simulink library "inp"  (R2021b)
settings: Solver=VariableStepAuto  StartTime=0.0  StopTime=10.0  RelTol=1e-3
undefined symbols (not defined in the file): C_TASK_5MS_S, FALSE, KINP_AcoreReadyToSlp_flg_ovrdflg, KINP_AcoreReadyToSlp_flg_ovrdval, KINP_AllowMovThd_OTA_enum_ovrdflg, KINP_AllowMovThd_OTA_enum_ovrdval, KINP_APSAngleTarget_Deg_ovrdflg, KINP_APSAngleTarget_Deg_ovrdval, KINP_APSDecReq_mps2_ovrdflg, KINP_APSDecReq_mps2_ovrdval, KINP_APSDecReqA_flg_ovrdflg, KINP_APSDecReqA_flg_ovrdval, KINP_APSDFLL_cm_ovrdflg, KINP_APSDFLL_cm_ovrdval, KINP_APSDFLR_cm_ovrdflg, KINP_APSDFLR_cm_ovrdval, KINP_APSDRLL_cm_ovrdflg, KINP_APSDRLL_cm_ovrdval, KINP_APSDRLR_cm_ovrdflg, KINP_APSDRLR_cm_ovrdval, KINP_APSExitCondition_enum_ovrdflg, KINP_APSExitCondition_enum_ovrdval, KINP_APSHWVer_enum_ovrdflg, KINP_APSHWVer_enum_ovrdval, KINP_APSProgressPCT_pct_ovrdflg, KINP_APSProgressPCT_pct_ovrdval, KINP_APSPwrReq_enum_ovrdflg, KINP_APSPwrReq_enum_ovrdval, KINP_APSReq_enum_ovrdflg, KINP_APSReq_enum_ovrdval, KINP_APSRQDisplay_enum_ovrdflg, KINP_APSRQDisplay_enum_ovrdval, KINP_APSRqEPASCtrl_flg_ovrdflg, KINP_APSRqEPASCtrl_flg_ovrdval, KINP_APSShiftPosnReq_enum_ovrdval, KINP_APSShiftPosnReq_enum_ovrflg, KINP_APSSpeedCMD_kph_ovrdval, KINP_APSSpeedCMD_kph_ovrflg, KINP_APSStaSystem_enum_ovrdflg, KINP_APSStaSystem_enum_ovrdval, KINP_APSSWVer_enum_ovrdflg, KINP_APSSWVer_enum_ovrdval, KINP_APSVMCReqA_flg_ovrdval, KINP_APSVMCReqA_flg_ovrflg, KINP_APSVRqEPASCtrl_flg_ovrdflg, KINP_APSVRqEPASCtrl_flg_ovrdval, KINP_AuxBattVolmV_mV_ovrdflg, KINP_AuxBattVolmV_mV_ovrdval, KINP_CAASSta_enum_ovrdflg, KINP_CAASSta_enum_ovrdval, KINP_CAASVMCReqA_flg_ovrdval, KINP_CAASVMCReqA_flg_ovrflg, KINP_CAN1BusOff_flg_ovrdflg, KINP_CAN1BusOff_flg_ovrdval, KINP_CAN2BusOff_flg_ovrdflg, KINP_CAN2BusOff_flg_ovrdval, KINP_CAN3BusOff_flg_ovrdflg, KINP_CAN3BusOff_flg_ovrdval, KINP_CAN4BusOff_flg_ovrdflg, KINP_CAN4BusOff_flg_ovrdval ... (+152)
libraries: FVT_lib x1035, hcu_lib x1
(part 8 of 33)

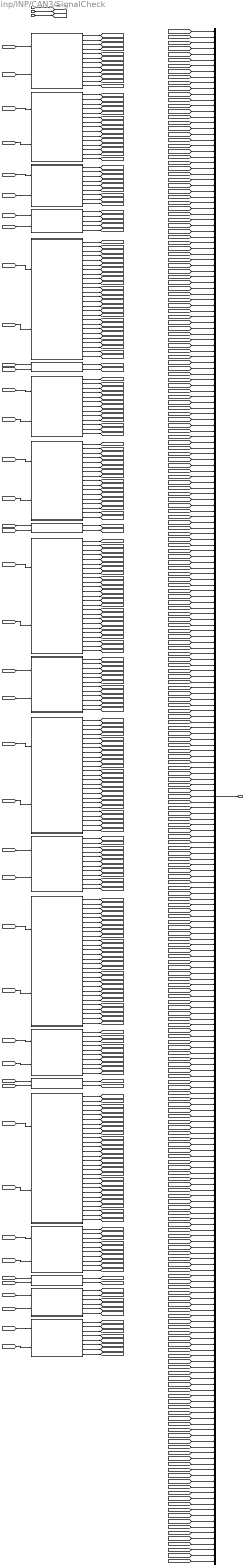
== system inp/INP/CAN3/SignalCheck ==
  inp_CanValid_bus : Inport
  TASK_TIME_S : Inport  Port=2
  BHAL_outputs : Inport  Port=3
  BMS1 : Subsystem
  BMS3 : Subsystem
  BMS4 : Subsystem
  BMS5 : Subsystem
  BMS6 : Subsystem
  BMS8 : Subsystem
  CCU1 : Subsystem
  CCU2 : Subsystem
  EBM1 : Subsystem
  MCU_B_F1 : Subsystem
  MCU_B_F2 : Subsystem
  MCU_B_R1 : Subsystem
  MCU_B_R2 : Subsystem
  MCU_N_F1 : Subsystem
  MCU_N_F2 : Subsystem
  MCU_N_F3 : Subsystem
  MCU_N_R1 : Subsystem
  MCU_N_R2 : Subsystem
  MCU_N_R3 : Subsystem
  Shifter1 : Subsystem
  Shifter2 : Subsystem
  bus_creator : BusCreator  Inputs=269
  inp_Hal_bus : Outport
  wires:
  inp_CanValid_bus/1 -> [inp_CanValid_bus]
  TASK_TIME_S/1 -> [TASK_TIME_S]
  BHAL_outputs/1 -> [BHAL_outputs]
  [BHAL_outputs] -> BMS1/1(BHAL_outputs)
  [inp_CanValid_bus] -> BMS1/2(inp_CanValid_bus)
  BMS1/1(VINP_BMS1CSErr_flg) -> [VINP_BMS1CSErr_flg]
  BMS1/2(VINP_BMS1RCErr_flg) -> [VINP_BMS1RCErr_flg]
  BMS1/3(VINP_BMSChckSum1_enum) -> [VINP_BMSChckSum1_enum]
  BMS1/4(VINP_BMSRolCnct1_enum) -> [VINP_BMSRolCnct1_enum]
  BMS1/5(VINP_HVBPwrAvailChrg_kW) -> [VINP_HVBPwrAvailChrg_kW]
  BMS1/6(VINP_HVBPwrAvailChrg30_kW) -> [VINP_HVBPwrAvailChrg30_kW]
  BMS1/7(VINP_HVBPwrAvailChrg60_kW) -> [VINP_HVBPwrAvailChrg60_kW]
  BMS1/8(VINP_HVBPwrAvailDchrg_kW) -> [VINP_HVBPwrAvailDchrg_kW]
  BMS1/9(VINP_HVBPwrAvailDchrg30_kW) -> [VINP_HVBPwrAvailDchrg30_kW]
  BMS1/10(VINP_HVBPwrAvailDchrg60_kW) -> [VINP_HVBPwrAvailDchrg60_kW]
  BMS1/11(VINP_HVBattCurr_A) -> [VINP_HVBattCurr_A]
  BMS1/12(VINP_HVBattVolt_V) -> [VINP_HVBattVolt_V]
  [BHAL_outputs] -> BMS3/1(BHAL_outputs)
  [inp_CanValid_bus] -> BMS3/2(inp_CanValid_bus)
  BMS3/1(VINP_ACChrgCurrDis_A) -> [VINP_ACChrgCurrDis_A]
  BMS3/2(VINP_FireDetErr_flg) -> [VINP_FireDetErr_flg]
  BMS3/3(VINP_HVBChrgPwr_kWh) -> [VINP_HVBChrgPwr_kWh]
  BMS3/4(VINP_HVBChrgPwrTotal_kWh) -> [VINP_HVBChrgPwrTotal_kWh]
  BMS3/5(VINP_HVBDrvPwr_kWh) -> [VINP_HVBDrvPwr_kWh]
  BMS3/6(VINP_HVBDrvPwrTotal_kWh) -> [VINP_HVBDrvPwrTotal_kWh]
  BMS3/7(VINP_HVBFullChrgPwr_kWh) -> [VINP_HVBFullChrgPwr_kWh]
  BMS3/8(VINP_HVBIsoImpedenceN_Megaohm) -> [VINP_HVBIsoImpedenceN_Megaohm]
  BMS3/9(VINP_HVBIsoImpedenceP_Megaohm) -> [VINP_HVBIsoImpedenceP_Megaohm]
  BMS3/10(VINP_HVBSOH_pct) -> [VINP_HVBSOH_pct]
  BMS3/11(VINP_HVBattErr_flg) -> [VINP_HVBattErr_flg]
  BMS3/12(VINP_HVBattPackVolt_V) -> [VINP_HVBattPackVolt_V]
  BMS3/13(VINP_HVBattSOC_pct) -> [VINP_HVBattSOC_pct]
  BMS3/14(VINP_HVBattSOCDis_pct) -> [VINP_HVBattSOCDis_pct]
  BMS3/15(VINP_RemainChrgTime_min) -> [VINP_RemainChrgTime_min]
  [BHAL_outputs] -> BMS4/1(BHAL_outputs)
  [inp_CanValid_bus] -> BMS4/2(inp_CanValid_bus)
  BMS4/1(VINP_CellTempAvg_C) -> [VINP_CellTempAvg_C]
  BMS4/2(VINP_HVBCellVoltMax_mV) -> [VINP_HVBCellVoltMax_mV]
  BMS4/3(VINP_HVBCellVoltMin_mV) -> [VINP_HVBCellVoltMin_mV]
  BMS4/4(VINP_HVBMTempMax_C) -> [VINP_HVBMTempMax_C]
  BMS4/5(VINP_HVBMTempMin_C) -> [VINP_HVBMTempMin_C]
  BMS4/6(VINP_MaxCellTempNum_enum) -> [VINP_MaxCellTempNum_enum]
  BMS4/7(VINP_MaxCellVoltNum_enum) -> [VINP_MaxCellVoltNum_enum]
  BMS4/8(VINP_MinCellTempNum_enum) -> [VINP_MinCellTempNum_enum]
  BMS4/9(VINP_MinCellVoltNum_enum) -> [VINP_MinCellVoltNum_enum]
  [BHAL_outputs] -> BMS5/1(BHAL_outputs)
  [inp_CanValid_bus] -> BMS5/2(inp_CanValid_bus)
  BMS5/1(VINP_HVInVolt_V) -> [VINP_HVInVolt_V]
  BMS5/2(VINP_LVBattDet12V_V) -> [VINP_LVBattDet12V_V]
  BMS5/3(VINP_OBCACCSLimit_A) -> [VINP_OBCACCSLimit_A]
  BMS5/4(VINP_OBCDCCurLm_A) -> [VINP_OBCDCCurLm_A]
  BMS5/5(VINP_OBCDCVoltLm_V) -> [VINP_OBCDCVoltLm_V]
  [BHAL_outputs] -> BMS6/1(BHAL_outputs)
  [inp_CanValid_bus] -> BMS6/2(inp_CanValid_bus)
  BMS6/1(VINP_BMS6CSErr_flg) -> [VINP_BMS6CSErr_flg]
  BMS6/2(VINP_BMS6RCErr_flg) -> [VINP_BMS6RCErr_flg]
  BMS6/3(VINP_BMSChckSum_enum) -> [VINP_BMSChckSum_enum]
  BMS6/4(VINP_BMSRolCnct_enum) -> [VINP_BMSRolCnct_enum]
  BMS6/5(VINP_BMSREADY_flg) -> [VINP_BMSREADY_flg]
  BMS6/6(VINP_BMSWarn1_flg) -> [VINP_BMSWarn1_flg]
  BMS6/7(VINP_BMSWarn2_flg) -> [VINP_BMSWarn2_flg]
  BMS6/8(VINP_BMSWarn3_flg) -> [VINP_BMSWarn3_flg]
  BMS6/9(VINP_BMSWarn4_flg) -> [VINP_BMSWarn4_flg]
  BMS6/10(VINP_BMSWarn5_flg) -> [VINP_BMSWarn5_flg]
  BMS6/11(VINP_BMSWarn6_flg) -> [VINP_BMSWarn6_flg]
  BMS6/12(VINP_BMSWarn7_flg) -> [VINP_BMSWarn7_flg]
  BMS6/13(VINP_BMSWarn8_flg) -> [VINP_BMSWarn8_flg]
  BMS6/14(VINP_ChrgInLockReq_enum) -> [VINP_ChrgInLockReq_enum]
  BMS6/15(VINP_ChrgPlugSta_enum) -> [VINP_ChrgPlugSta_enum]
  BMS6/16(VINP_DisChrgPlugErr_enum) -> [VINP_DisChrgPlugErr_enum]
  BMS6/17(VINP_ExtChrgSta_enum) -> [VINP_ExtChrgSta_enum]
  BMS6/18(VINP_HVBChrgErr_enum) -> [VINP_HVBChrgErr_enum]
  BMS6/19(VINP_HVBContactorSta_flg) -> [VINP_HVBContactorSta_flg]
  BMS6/20(VINP_HVBHVILErr_flg) -> [VINP_HVBHVILErr_flg]
  BMS6/21(VINP_HVBOvrTempErr_flg) -> [VINP_HVBOvrTempErr_flg]
  BMS6/22(VINP_HVBOvrTempWarn_enum) -> [VINP_HVBOvrTempWarn_enum]
  BMS6/23(VINP_HVBPreheatPrecoolSta_enum) -> [VINP_HVBPreheatPrecoolSta_enum]
  BMS6/24(VINP_HVBattReady4Pre_enum) -> [VINP_HVBattReady4Pre_enum]
  BMS6/25(VINP_HVILSta_flg) -> [VINP_HVILSta_flg]
  BMS6/26(VINP_V2LSta_enum) -> [VINP_V2LSta_enum]
  [BHAL_outputs] -> BMS8/1(BHAL_outputs)
  [inp_CanValid_bus] -> BMS8/2(inp_CanValid_bus)
  BMS8/1(VINP_MainRlyNegSta_enum) -> [VINP_MainRlyNegSta_enum]
  BMS8/2(VINP_MainRlyPosSta_enum) -> [VINP_MainRlyPosSta_enum]
  [BHAL_outputs] -> CCU1/1(BHAL_outputs)
  [inp_CanValid_bus] -> CCU1/2(inp_CanValid_bus)
  CCU1/1(VINP_CCU1CSErr_flg) -> [VINP_CCU1CSErr_flg]
  CCU1/2(VINP_CCU1RCErr_flg) -> [VINP_CCU1RCErr_flg]
  CCU1/3(VINP_CSCCU1_enum) -> [VINP_CSCCU1_enum]
  CCU1/4(VINP_DCDCAuxCur_A) -> [VINP_DCDCAuxCur_A]
  CCU1/5(VINP_DCDCAuxVolt_V) -> [VINP_DCDCAuxVolt_V]
  CCU1/6(VINP_DCDCHVCur_A) -> [VINP_DCDCHVCur_A]
  CCU1/7(VINP_DCDCInVoltInf_V) -> [VINP_DCDCInVoltInf_V]
  CCU1/8(VINP_DCDCPreCompleted_enum) -> [VINP_DCDCPreCompleted_enum]
  CCU1/9(VINP_OBCDCCurrInf_A) -> [VINP_OBCDCCurrInf_A]
  CCU1/10(VINP_OBCDCVoltInf_V) -> [VINP_OBCDCVoltInf_V]
  CCU1/11(VINP_OBCPreCompleted_enum) -> [VINP_OBCPreCompleted_enum]
  CCU1/12(VINP_OBCWakeup4Plugin_flg) -> [VINP_OBCWakeup4Plugin_flg]
  CCU1/13(VINP_RCCCU1_enum) -> [VINP_RCCCU1_enum]
  [BHAL_outputs] -> CCU2/1(BHAL_outputs)
  [inp_CanValid_bus] -> CCU2/2(inp_CanValid_bus)
  CCU2/1(VINP_CCU2CSErr_flg) -> [VINP_CCU2CSErr_flg]
  CCU2/2(VINP_CCU2RCErr_flg) -> [VINP_CCU2RCErr_flg]
  CCU2/3(VINP_CSCCU2_enum) -> [VINP_CSCCU2_enum]
  CCU2/4(VINP_DCDCEnaSta_flg) -> [VINP_DCDCEnaSta_flg]
  CCU2/5(VINP_DCDCFaultSta_enum) -> [VINP_DCDCFaultSta_enum]
  CCU2/6(VINP_DCDCReady4Pre_flg) -> [VINP_DCDCReady4Pre_flg]
  CCU2/7(VINP_DCDCTemp_C) -> [VINP_DCDCTemp_C]
  CCU2/8(VINP_OBCACCurrInf_A) -> [VINP_OBCACCurrInf_A]
  CCU2/9(VINP_OBCACVoltInf_V) -> [VINP_OBCACVoltInf_V]
  CCU2/10(VINP_OBCEnaSta_flg) -> [VINP_OBCEnaSta_flg]
  CCU2/11(VINP_OBCFaultSta_enum) -> [VINP_OBCFaultSta_enum]
  CCU2/12(VINP_OBCPluginSta_flg) -> [VINP_OBCPluginSta_flg]
  CCU2/13(VINP_OBCReady4Pre_flg) -> [VINP_OBCReady4Pre_flg]
  CCU2/14(VINP_OBCTemp_C) -> [VINP_OBCTemp_C]
  CCU2/15(VINP_OBCV2LSta_enum) -> [VINP_OBCV2LSta_enum]
  CCU2/16(VINP_OBCACCurLim_enum) -> [VINP_OBCACCurLim_enum]
  CCU2/17(VINP_RCCCU2_enum) -> [VINP_RCCCU2_enum]
  [BHAL_outputs] -> EBM1/1(BHAL_outputs)
  [inp_CanValid_bus] -> EBM1/2(inp_CanValid_bus)
  EBM1/1(VINP_EBMErrSta_enum) -> [VINP_EBMErrSta_enum]
  EBM1/2(VINP_EBMRLampSta_enum) -> [VINP_EBMRLampSta_enum]
  [BHAL_outputs] -> MCU_B_F1/1(BHAL_outputs)
  [inp_CanValid_bus] -> MCU_B_F1/2(inp_CanValid_bus)
  MCU_B_F1/1(VINP_FrActvDmpDisabSta_flg) -> [VINP_FrActvDmpDisabSta_flg]
  MCU_B_F1/2(VINP_FrEDUDrtSta_flg) -> [VINP_FrEDUDrtSta_flg]
  MCU_B_F1/3(VINP_FrEDUOpratingSta_flg) -> [VINP_FrEDUOpratingSta_flg]
  MCU_B_F1/4(VINP_FrEDURealTMTq_Nm) -> [VINP_FrEDURealTMTq_Nm]
  MCU_B_F1/5(VINP_FrEDURotateDirction_enum) -> [VINP_FrEDURotateDirction_enum]
  MCU_B_F1/6(VINP_FrEDUTqReqFbk_Nm) -> [VINP_FrEDUTqReqFbk_Nm]
  MCU_B_F1/7(VINP_FrMCUBAT_V) -> [VINP_FrMCUBAT_V]
  MCU_B_F1/8(VINP_FrMCUDCBusCurr_A) -> [VINP_FrMCUDCBusCurr_A]
  MCU_B_F1/9(VINP_FrMCUDCBusVolt_V) -> [VINP_FrMCUDCBusVolt_V]
  MCU_B_F1/10(VINP_FrMCUDischrgSta_flg) -> [VINP_FrMCUDischrgSta_flg]
  MCU_B_F1/11(VINP_FrMCUEnaSta_flg) -> [VINP_FrMCUEnaSta_flg]
  MCU_B_F1/12(VINP_FrMCUErr_enum) -> [VINP_FrMCUErr_enum]
  MCU_B_F1/13(VINP_FrMCUIGNsta_flg) -> [VINP_FrMCUIGNsta_flg]
  MCU_B_F1/14(VINP_FrMCUReady_flg) -> [VINP_FrMCUReady_flg]
  MCU_B_F1/15(VINP_FrMCUReady4Pre_flg) -> [VINP_FrMCUReady4Pre_flg]
  MCU_B_F1/16(VINP_FrMCUSysSta_enum) -> [VINP_FrMCUSysSta_enum]
  MCU_B_F1/17(VINP_FrMCUTemp_C) -> [VINP_FrMCUTemp_C]
  MCU_B_F1/18(VINP_FrMotorAvailTq_Nm) -> [VINP_FrMotorAvailTq_Nm]
  MCU_B_F1/19(VINP_FrRegenAvailTq_Nm) -> [VINP_FrRegenAvailTq_Nm]
  MCU_B_F1/20(VINP_FrTMSpd_rpm) -> [VINP_FrTMSpd_rpm]
  MCU_B_F1/21(VINP_FrTMTemp_C) -> [VINP_FrTMTemp_C]
  MCU_B_F1/22(VINP_FrTMid_A) -> [VINP_FrTMid_A]
  MCU_B_F1/23(VINP_FrTMiq_A) -> [VINP_FrTMiq_A]
  MCU_B_F1/24(VINP_MCUWarnF_enum) -> [VINP_MCUWarnF_enum]
  MCU_B_F1/25(VINP_MCUBFRealPwrKwSta_kW) -> [VINP_MCUBFRealPwrKwSta_kW]
  [BHAL_outputs] -> MCU_B_F2/1(BHAL_outputs)
  [inp_CanValid_bus] -> MCU_B_F2/2(inp_CanValid_bus)
  MCU_B_F2/1(VINP_FrCoolanttempReq_C) -> [VINP_FrCoolanttempReq_C]
  MCU_B_F2/2(VINP_FrFailcode1_enum) -> [VINP_FrFailcode1_enum]
  MCU_B_F2/3(VINP_FrFailcode2_enum) -> [VINP_FrFailcode2_enum]
  MCU_B_F2/4(VINP_FrFailcodehistory1_enum) -> [VINP_FrFailcodehistory1_enum]
  MCU_B_F2/5(VINP_FrFailcodehistory2_enum) -> [VINP_FrFailcodehistory2_enum]
  MCU_B_F2/6(VINP_FrLLCTemp_C) -> [VINP_FrLLCTemp_C]
  MCU_B_F2/7(VINP_FrLLCflowReq_Lpmin) -> [VINP_FrLLCflowReq_Lpmin]
  MCU_B_F2/8(VINP_FrMCUTempWarn_enum) -> [VINP_FrMCUTempWarn_enum]
  MCU_B_F2/9(VINP_FrMCUHWVer_enum) -> [VINP_FrMCUHWVer_enum]
  MCU_B_F2/10(VINP_FrMCUSWVer_enum) -> [VINP_FrMCUSWVer_enum]
  MCU_B_F2/11(VINP_FrTMTempWarn_enum) -> [VINP_FrTMTempWarn_enum]
  MCU_B_F2/12(VINP_MCUBFLLCTempWarnSta_enum) -> [VINP_MCUBFLLCTempWarnSta_enum]
  [BHAL_outputs] -> MCU_B_R1/1(BHAL_outputs)
  [inp_CanValid_bus] -> MCU_B_R1/2(inp_CanValid_bus)
  MCU_B_R1/1(VINP_MCUWarnR_enum) -> [VINP_MCUWarnR_enum]
  MCU_B_R1/2(VINP_MCUBRRealPwrKwSta_kW) -> [VINP_MCUBRRealPwrKwSta_kW]
  MCU_B_R1/3(VINP_RrActvDmpDisabSta_flg) -> [VINP_RrActvDmpDisabSta_flg]
  MCU_B_R1/4(VINP_RrEDUDrtSta_flg) -> [VINP_RrEDUDrtSta_flg]
  MCU_B_R1/5(VINP_RrEDUOpratingSta_flg) -> [VINP_RrEDUOpratingSta_flg]
  MCU_B_R1/6(VINP_RrEDURealTMTq_Nm) -> [VINP_RrEDURealTMTq_Nm]
  MCU_B_R1/7(VINP_RrEDURotateDirction_enum) -> [VINP_RrEDURotateDirction_enum]
  MCU_B_R1/8(VINP_RrEDUTqReqFbk_Nm) -> [VINP_RrEDUTqReqFbk_Nm]
  MCU_B_R1/9(VINP_RrMCUBAT_V) -> [VINP_RrMCUBAT_V]
  MCU_B_R1/10(VINP_RrMCUDCBusCurr_A) -> [VINP_RrMCUDCBusCurr_A]
  MCU_B_R1/11(VINP_RrMCUDCBusVolt_V) -> [VINP_RrMCUDCBusVolt_V]
  MCU_B_R1/12(VINP_RrMCUDischrgSta_flg) -> [VINP_RrMCUDischrgSta_flg]
  MCU_B_R1/13(VINP_RrMCUEnaSta_flg) -> [VINP_RrMCUEnaSta_flg]
  MCU_B_R1/14(VINP_RrMCUErr_enum) -> [VINP_RrMCUErr_enum]
  MCU_B_R1/15(VINP_RrMCUIGNsta_flg) -> [VINP_RrMCUIGNsta_flg]
  MCU_B_R1/16(VINP_RrMCUReady_flg) -> [VINP_RrMCUReady_flg]
  MCU_B_R1/17(VINP_RrMCUReady4Pre_flg) -> [VINP_RrMCUReady4Pre_flg]
  MCU_B_R1/18(VINP_RrMCUSysSta_enum) -> [VINP_RrMCUSysSta_enum]
  MCU_B_R1/19(VINP_RrMCUTemp_C) -> [VINP_RrMCUTemp_C]
  MCU_B_R1/20(VINP_RrMotorAvailTq_Nm) -> [VINP_RrMotorAvailTq_Nm]
  MCU_B_R1/21(VINP_RrRegenAvailTq_Nm) -> [VINP_RrRegenAvailTq_Nm]
  MCU_B_R1/22(VINP_RrTMSpd_rpm) -> [VINP_RrTMSpd_rpm]
  MCU_B_R1/23(VINP_RrTMTemp_C) -> [VINP_RrTMTemp_C]
  MCU_B_R1/24(VINP_RrTMid_A) -> [VINP_RrTMid_A]
  MCU_B_R1/25(VINP_RrTMiq_A) -> [VINP_RrTMiq_A]
  [BHAL_outputs] -> MCU_B_R2/1(BHAL_outputs)
  [inp_CanValid_bus] -> MCU_B_R2/2(inp_CanValid_bus)
  MCU_B_R2/1(VINP_MCUBRLLCTempWarnSta_enum) -> [VINP_MCUBRLLCTempWarnSta_enum]
  MCU_B_R2/2(VINP_RrCoolanttempReq_cnt) -> [VINP_RrCoolanttempReq_cnt]
  MCU_B_R2/3(VINP_RrFailcode1_enum) -> [VINP_RrFailcode1_enum]
  MCU_B_R2/4(VINP_RrFailcode2_enum) -> [VINP_RrFailcode2_enum]
  MCU_B_R2/5(VINP_RrFailcodehistory1_enum) -> [VINP_RrFailcodehistory1_enum]
  MCU_B_R2/6(VINP_RrFailcodehistory2_enum) -> [VINP_RrFailcodehistory2_enum]
  MCU_B_R2/7(VINP_RrLLCTemp_C) -> [VINP_RrLLCTemp_C]
  MCU_B_R2/8(VINP_RrLLCflowReq_Lpmin) -> [VINP_RrLLCflowReq_Lpmin]
  MCU_B_R2/9(VINP_RrMCU3HWVer_enum) -> [VINP_RrMCU3HWVer_enum]
  MCU_B_R2/10(VINP_RrMCU3SWVer_enum) -> [VINP_RrMCU3SWVer_enum]
  MCU_B_R2/11(VINP_RrMCUTempWarn_enum) -> [VINP_RrMCUTempWarn_enum]
  MCU_B_R2/12(VINP_RrTMTempWarn_enum) -> [VINP_RrTMTempWarn_enum]
  [BHAL_outputs] -> MCU_N_F1/1(BHAL_outputs)
  [inp_CanValid_bus] -> MCU_N_F1/2(inp_CanValid_bus)
  MCU_N_F1/1(VINP_MCUNF1CSErr_flg) -> [VINP_MCUNF1CSErr_flg]
  MCU_N_F1/2(VINP_MCUNF1RCErr_flg) -> [VINP_MCUNF1RCErr_flg]
  MCU_N_F1/3(VINP_FrActvDmpDisabStaNidec_flg) -> [VINP_FrActvDmpDisabStaNidec_flg]
  MCU_N_F1/4(VINP_FrEDUDrtStaNidec_flg) -> [VINP_FrEDUDrtStaNidec_flg]
  MCU_N_F1/5(VINP_FrEDUOpratingStaNidec_flg) -> [VINP_FrEDUOpratingStaNidec_flg]
  MCU_N_F1/6(VINP_FrEDURealTMTqNidec_Nm) -> [VINP_FrEDURealTMTqNidec_Nm]
  MCU_N_F1/7(VINP_FrEDURotateDirctionNidec_enum) -> [VINP_FrEDURotateDirctionNidec_enum]
  MCU_N_F1/8(VINP_FrEDUTqReqFbkNidec_Nm) -> [VINP_FrEDUTqReqFbkNidec_Nm]
  MCU_N_F1/9(VINP_FrMCU1ChksumNidec_enum) -> [VINP_FrMCU1ChksumNidec_enum]
  MCU_N_F1/10(VINP_FrMCU1RolCntNidec_enum) -> [VINP_FrMCU1RolCntNidec_enum]
  MCU_N_F1/11(VINP_FrMCUBATNidec_V) -> [VINP_FrMCUBATNidec_V]
  MCU_N_F1/12(VINP_FrMCUDCBusCurrNidec_A) -> [VINP_FrMCUDCBusCurrNidec_A]
  MCU_N_F1/13(VINP_FrMCUDCBusVoltNidec_V) -> [VINP_FrMCUDCBusVoltNidec_V]
  MCU_N_F1/14(VINP_FrMCUDischrgStaNidec_flg) -> [VINP_FrMCUDischrgStaNidec_flg]
  MCU_N_F1/15(VINP_FrMCUEnaStaNidec_flg) -> [VINP_FrMCUEnaStaNidec_flg]
  MCU_N_F1/16(VINP_FrMCUErrNidec_enum) -> [VINP_FrMCUErrNidec_enum]
  MCU_N_F1/17(VINP_FrMCUIGNstaNidec_flg) -> [VINP_FrMCUIGNstaNidec_flg]
  MCU_N_F1/18(VINP_FrMCUReady4PreNidec_flg) -> [VINP_FrMCUReady4PreNidec_flg]
  MCU_N_F1/19(VINP_FrMCUReadyNidec_flg) -> [VINP_FrMCUReadyNidec_flg]
  MCU_N_F1/20(VINP_FrMCUSysStaNidec_enum) -> [VINP_FrMCUSysStaNidec_enum]
  MCU_N_F1/21(VINP_FrMCUTempNidec_C) -> [VINP_FrMCUTempNidec_C]
  MCU_N_F1/22(VINP_FrMotorAvailTqNidec_Nm) -> [VINP_FrMotorAvailTqNidec_Nm]
  MCU_N_F1/23(VINP_FrRegenAvailTqNidec_Nm) -> [VINP_FrRegenAvailTqNidec_Nm]
  MCU_N_F1/24(VINP_FrTMSpdNidec_rpm) -> [VINP_FrTMSpdNidec_rpm]
  MCU_N_F1/25(VINP_FrTMTempNidec_C) -> [VINP_FrTMTempNidec_C]
  MCU_N_F1/26(VINP_FrTMidNidec_A) -> [VINP_FrTMidNidec_A]
  MCU_N_F1/27(VINP_FrTMiqNidec_A) -> [VINP_FrTMiqNidec_A]
  MCU_N_F1/28(VINP_MCUWarnFNidec_enum) -> [VINP_MCUWarnFNidec_enum]
  [BHAL_outputs] -> MCU_N_F2/1(BHAL_outputs)
  [inp_CanValid_bus] -> MCU_N_F2/2(inp_CanValid_bus)
  MCU_N_F2/1(VINP_FrCoolanttempReqNidec_C) -> [VINP_FrCoolanttempReqNidec_C]
  MCU_N_F2/2(VINP_FrEOPSpdSetNidec_rpm) -> [VINP_FrEOPSpdSetNidec_rpm]
  MCU_N_F2/3(VINP_FrFailcode1Nidec_enum) -> [VINP_FrFailcode1Nidec_enum]
  MCU_N_F2/4(VINP_FrFailcode2Nidec_enum) -> [VINP_FrFailcode2Nidec_enum]
  MCU_N_F2/5(VINP_FrFailcodehistory1Nidec_enum) -> [VINP_FrFailcodehistory1Nidec_enum]
  MCU_N_F2/6(VINP_FrFailcodehistory2Nidec_enum) -> [VINP_FrFailcodehistory2Nidec_enum]
  MCU_N_F2/7(VINP_FrLLCTempNidec_C) -> [VINP_FrLLCTempNidec_C]
  MCU_N_F2/8(VINP_FrLLCflowReqNidec_Lpmin) -> [VINP_FrLLCflowReqNidec_Lpmin]
  MCU_N_F2/9(VINP_FrMCUTempWarnNidec_enum) -> [VINP_FrMCUTempWarnNidec_enum]
  MCU_N_F2/10(VINP_FrTMTempWarnNidec_enum) -> [VINP_FrTMTempWarnNidec_enum]
  [BHAL_outputs] -> MCU_N_F3/1(BHAL_outputs)
  [inp_CanValid_bus] -> MCU_N_F3/2(inp_CanValid_bus)
  MCU_N_F3/1(VINP_FrMCUHWVerNidec_enum) -> [VINP_FrMCUHWVerNidec_enum]
  MCU_N_F3/2(VINP_FrMCUSWVerNidec_enum) -> [VINP_FrMCUSWVerNidec_enum]
  [BHAL_outputs] -> MCU_N_R1/1(BHAL_outputs)
  [inp_CanValid_bus] -> MCU_N_R1/2(inp_CanValid_bus)
  MCU_N_R1/1(VINP_MCUNR1CSErr_flg) -> [VINP_MCUNR1CSErr_flg]
  MCU_N_R1/2(VINP_MCUNR1RCErr_flg) -> [VINP_MCUNR1RCErr_flg]
  MCU_N_R1/3(VINP_MCUWarnRNidec_enum) -> [VINP_MCUWarnRNidec_enum]
  MCU_N_R1/4(VINP_RrActvDmpDisabStaNidec_flg) -> [VINP_RrActvDmpDisabStaNidec_flg]
  MCU_N_R1/5(VINP_RrEDUDrtStaNidec_flg) -> [VINP_RrEDUDrtStaNidec_flg]
  MCU_N_R1/6(VINP_RrEDUOpratingStaNidec_flg) -> [VINP_RrEDUOpratingStaNidec_flg]
  MCU_N_R1/7(VINP_RrEDURealTMTqNidec_Nm) -> [VINP_RrEDURealTMTqNidec_Nm]
  MCU_N_R1/8(VINP_RrEDURotateDirctionNidec_enum) -> [VINP_RrEDURotateDirctionNidec_enum]
  MCU_N_R1/9(VINP_RrEDUTqReqFbkNidec_Nm) -> [VINP_RrEDUTqReqFbkNidec_Nm]
  MCU_N_R1/10(VINP_RrMCU1ChksumNidec_enum) -> [VINP_RrMCU1ChksumNidec_enum]
  MCU_N_R1/11(VINP_RrMCU1RolCntNidec_enum) -> [VINP_RrMCU1RolCntNidec_enum]
  MCU_N_R1/12(VINP_RrMCUBATNidec_V) -> [VINP_RrMCUBATNidec_V]
  MCU_N_R1/13(VINP_RrMCUDCBusCurrNidec_A) -> [VINP_RrMCUDCBusCurrNidec_A]
  MCU_N_R1/14(VINP_RrMCUDCBusVoltNidec_V) -> [VINP_RrMCUDCBusVoltNidec_V]
  MCU_N_R1/15(VINP_RrMCUDischrgStaNidec_flg) -> [VINP_RrMCUDischrgStaNidec_flg]
  MCU_N_R1/16(VINP_RrMCUEnaStaNidec_flg) -> [VINP_RrMCUEnaStaNidec_flg]
  MCU_N_R1/17(VINP_RrMCUErrNidec_enum) -> [VINP_RrMCUErrNidec_enum]
  MCU_N_R1/18(VINP_RrMCUIGNstaNidec_flg) -> [VINP_RrMCUIGNstaNidec_flg]
  MCU_N_R1/19(VINP_RrMCUReady4PreNidec_flg) -> [VINP_RrMCUReady4PreNidec_flg]
  MCU_N_R1/20(VINP_RrMCUReadyNidec_flg) -> [VINP_RrMCUReadyNidec_flg]
  MCU_N_R1/21(VINP_RrMCUSysStaNidec_enum) -> [VINP_RrMCUSysStaNidec_enum]
  MCU_N_R1/22(VINP_RrMCUTempNidec_C) -> [VINP_RrMCUTempNidec_C]
  MCU_N_R1/23(VINP_RrMotorAvailTqNidec_Nm) -> [VINP_RrMotorAvailTqNidec_Nm]
  MCU_N_R1/24(VINP_RrRegenAvailTqNidec_Nm) -> [VINP_RrRegenAvailTqNidec_Nm]
  MCU_N_R1/25(VINP_RrTMSpdNidec_rpm) -> [VINP_RrTMSpdNidec_rpm]
  MCU_N_R1/26(VINP_RrTMTempNidec_C) -> [VINP_RrTMTempNidec_C]
  MCU_N_R1/27(VINP_RrTMidNidec_A) -> [VINP_RrTMidNidec_A]
  MCU_N_R1/28(VINP_RrTMiqNidec_A) -> [VINP_RrTMiqNidec_A]
  [BHAL_outputs] -> MCU_N_R2/1(BHAL_outputs)
  [inp_CanValid_bus] -> MCU_N_R2/2(inp_CanValid_bus)
  MCU_N_R2/1(VINP_RrCoolanttempReqNidec_cnt) -> [VINP_RrCoolanttempReqNidec_cnt]
  MCU_N_R2/2(VINP_RrEOPSpdSetNidec_rpm) -> [VINP_RrEOPSpdSetNidec_rpm]
  MCU_N_R2/3(VINP_RrFailcode1Nidec_enum) -> [VINP_RrFailcode1Nidec_enum]
  MCU_N_R2/4(VINP_RrFailcode2Nidec_enum) -> [VINP_RrFailcode2Nidec_enum]
  MCU_N_R2/5(VINP_RrFailcodehistory1Nidec_enum) -> [VINP_RrFailcodehistory1Nidec_enum]
  MCU_N_R2/6(VINP_RrFailcodehistory2Nidec_enum) -> [VINP_RrFailcodehistory2Nidec_enum]
  MCU_N_R2/7(VINP_RrLLCTempNidec_C) -> [VINP_RrLLCTempNidec_C]
  MCU_N_R2/8(VINP_RrLLCflowReqNidec_Lpmin) -> [VINP_RrLLCflowReqNidec_Lpmin]
  MCU_N_R2/9(VINP_RrMCUTempWarnNidec_enum) -> [VINP_RrMCUTempWarnNidec_enum]
  MCU_N_R2/10(VINP_RrTMTempWarnNidec_enum) -> [VINP_RrTMTempWarnNidec_enum]
  [BHAL_outputs] -> MCU_N_R3/1(BHAL_outputs)
  [inp_CanValid_bus] -> MCU_N_R3/2(inp_CanValid_bus)
  MCU_N_R3/1(VINP_RrMCU3HWVerNidec_enum) -> [VINP_RrMCU3HWVerNidec_enum]
  MCU_N_R3/2(VINP_RrMCU3SWVerNidec_enum) -> [VINP_RrMCU3SWVerNidec_enum]
  [BHAL_outputs] -> Shifter1/1(BHAL_outputs)
  [inp_CanValid_bus] -> Shifter1/2(inp_CanValid_bus)
  Shifter1/1(VINP_Shifter1CSErr_flg) -> [VINP_Shifter1CSErr_flg]
  Shifter1/2(VINP_Shifter1RCErr_flg) -> [VINP_Shifter1RCErr_flg]
  Shifter1/3(VINP_ShifterCRC8_enum) -> [VINP_ShifterCRC8_enum]
  Shifter1/4(VINP_ShifterFailsta_enum) -> [VINP_ShifterFailsta_enum]
  Shifter1/5(VINP_ShifterHandleCmd_enum) -> [VINP_ShifterHandleCmd_enum]
  Shifter1/6(VINP_ShifterRC_enum) -> [VINP_ShifterRC_enum]
  [BHAL_outputs] -> Shifter2/1(BHAL_outputs)
  [inp_CanValid_bus] -> Shifter2/2(inp_CanValid_bus)
  Shifter2/1(VINP_Shifter2CSErr_flg) -> [VINP_Shifter2CSErr_flg]
  Shifter2/2(VINP_Shifter2RCErr_flg) -> [VINP_Shifter2RCErr_flg]
  Shifter2/3(VINP_CSW2DimSwSta_flg) -> [VINP_CSW2DimSwSta_flg]
  Shifter2/4(VINP_CSW2FWasSwSta_enum) -> [VINP_CSW2FWasSwSta_enum]
  Shifter2/5(VINP_CSW2FWipSwSta_enum) -> [VINP_CSW2FWipSwSta_enum]
  Shifter2/6(VINP_CSW2PassSWSta_flg) -> [VINP_CSW2PassSWSta_flg]
  Shifter2/7(VINP_CSW2RWipWasSwSta_enum) -> [VINP_CSW2RWipWasSwSta_enum]
  Shifter2/8(VINP_CSW2TurnSwSta_enum) -> [VINP_CSW2TurnSwSta_enum]
  bus_creator/1 -> inp_Hal_bus/1
  [VINP_BMS1CSErr_flg] -> bus_creator/1
  [VINP_BMS1RCErr_flg] -> bus_creator/2
  [VINP_BMSChckSum1_enum] -> bus_creator/3
  [VINP_BMSRolCnct1_enum] -> bus_creator/4
  [VINP_HVBPwrAvailChrg_kW] -> bus_creator/5
  [VINP_HVBPwrAvailChrg30_kW] -> bus_creator/6
  [VINP_HVBPwrAvailChrg60_kW] -> bus_creator/7
  [VINP_HVBPwrAvailDchrg_kW] -> bus_creator/8
  [VINP_HVBPwrAvailDchrg30_kW] -> bus_creator/9
  [VINP_HVBPwrAvailDchrg60_kW] -> bus_creator/10
  [VINP_HVBattCurr_A] -> bus_creator/11
  [VINP_HVBattVolt_V] -> bus_creator/12
  [VINP_ACChrgCurrDis_A] -> bus_creator/13
  [VINP_FireDetErr_flg] -> bus_creator/14
  [VINP_HVBChrgPwr_kWh] -> bus_creator/15
  [VINP_HVBChrgPwrTotal_kWh] -> bus_creator/16
  [VINP_HVBDrvPwr_kWh] -> bus_creator/17
  [VINP_HVBDrvPwrTotal_kWh] -> bus_creator/18
  [VINP_HVBFullChrgPwr_kWh] -> bus_creator/19
  [VINP_HVBIsoImpedenceN_Megaohm] -> bus_creator/20
  [VINP_HVBIsoImpedenceP_Megaohm] -> bus_creator/21
  [VINP_HVBSOH_pct] -> bus_creator/22
  [VINP_HVBattErr_flg] -> bus_creator/23
  [VINP_HVBattPackVolt_V] -> bus_creator/24
  [VINP_HVBattSOC_pct] -> bus_creator/25
  [VINP_HVBattSOCDis_pct] -> bus_creator/26
  [VINP_RemainChrgTime_min] -> bus_creator/27
  [VINP_CellTempAvg_C] -> bus_creator/28
  [VINP_HVBCellVoltMax_mV] -> bus_creator/29
  [VINP_HVBCellVoltMin_mV] -> bus_creator/30
  [VINP_HVBMTempMax_C] -> bus_creator/31
  [VINP_HVBMTempMin_C] -> bus_creator/32
  [VINP_MaxCellTempNum_enum] -> bus_creator/33
  [VINP_MaxCellVoltNum_enum] -> bus_creator/34
  [VINP_MinCellTempNum_enum] -> bus_creator/35
  [VINP_MinCellVoltNum_enum] -> bus_creator/36
  [VINP_HVInVolt_V] -> bus_creator/37
  [VINP_LVBattDet12V_V] -> bus_creator/38
  [VINP_OBCACCSLimit_A] -> bus_creator/39
  [VINP_OBCDCCurLm_A] -> bus_creator/40
  [VINP_OBCDCVoltLm_V] -> bus_creator/41
  [VINP_BMS6CSErr_flg] -> bus_creator/42
  [VINP_BMS6RCErr_flg] -> bus_creator/43
  [VINP_BMSChckSum_enum] -> bus_creator/44
  [VINP_BMSRolCnct_enum] -> bus_creator/45
  [VINP_BMSREADY_flg] -> bus_creator/46
  [VINP_BMSWarn1_flg] -> bus_creator/47
  [VINP_BMSWarn2_flg] -> bus_creator/48
  [VINP_BMSWarn3_flg] -> bus_creator/49
  [VINP_BMSWarn4_flg] -> bus_creator/50
  [VINP_BMSWarn5_flg] -> bus_creator/51
  [VINP_BMSWarn6_flg] -> bus_creator/52
  [VINP_BMSWarn7_flg] -> bus_creator/53
  [VINP_BMSWarn8_flg] -> bus_creator/54
  [VINP_ChrgInLockReq_enum] -> bus_creator/55
  [VINP_ChrgPlugSta_enum] -> bus_creator/56
  [VINP_DisChrgPlugErr_enum] -> bus_creator/57
  [VINP_ExtChrgSta_enum] -> bus_creator/58
  [VINP_HVBChrgErr_enum] -> bus_creator/59
  [VINP_HVBContactorSta_flg] -> bus_creator/60
  [VINP_HVBHVILErr_flg] -> bus_creator/61
  [VINP_HVBOvrTempErr_flg] -> bus_creator/62
  [VINP_HVBOvrTempWarn_enum] -> bus_creator/63
  [VINP_HVBPreheatPrecoolSta_enum] -> bus_creator/64
  [VINP_HVBattReady4Pre_enum] -> bus_creator/65
  [VINP_HVILSta_flg] -> bus_creator/66
  [VINP_V2LSta_enum] -> bus_creator/67
  [VINP_MainRlyNegSta_enum] -> bus_creator/68
  [VINP_MainRlyPosSta_enum] -> bus_creator/69
  [VINP_CCU1CSErr_flg] -> bus_creator/70
  [VINP_CCU1RCErr_flg] -> bus_creator/71
  [VINP_CSCCU1_enum] -> bus_creator/72
  [VINP_DCDCAuxCur_A] -> bus_creator/73
  [VINP_DCDCAuxVolt_V] -> bus_creator/74
  [VINP_DCDCHVCur_A] -> bus_creator/75
  [VINP_DCDCInVoltInf_V] -> bus_creator/76
  [VINP_DCDCPreCompleted_enum] -> bus_creator/77
  [VINP_OBCDCCurrInf_A] -> bus_creator/78
  [VINP_OBCDCVoltInf_V] -> bus_creator/79
  [VINP_OBCPreCompleted_enum] -> bus_creator/80
  [VINP_OBCWakeup4Plugin_flg] -> bus_creator/81
  [VINP_RCCCU1_enum] -> bus_creator/82
  [VINP_CCU2CSErr_flg] -> bus_creator/83
  [VINP_CCU2RCErr_flg] -> bus_creator/84
  [VINP_CSCCU2_enum] -> bus_creator/85
  [VINP_DCDCEnaSta_flg] -> bus_creator/86
  [VINP_DCDCFaultSta_enum] -> bus_creator/87
  [VINP_DCDCReady4Pre_flg] -> bus_creator/88
  [VINP_DCDCTemp_C] -> bus_creator/89
  [VINP_OBCACCurrInf_A] -> bus_creator/90
  [VINP_OBCACVoltInf_V] -> bus_creator/91
  [VINP_OBCEnaSta_flg] -> bus_creator/92
  [VINP_OBCFaultSta_enum] -> bus_creator/93
  [VINP_OBCPluginSta_flg] -> bus_creator/94
  [VINP_OBCReady4Pre_flg] -> bus_creator/95
  [VINP_OBCTemp_C] -> bus_creator/96
  [VINP_OBCV2LSta_enum] -> bus_creator/97
  [VINP_OBCACCurLim_enum] -> bus_creator/98
  [VINP_RCCCU2_enum] -> bus_creator/99
  [VINP_EBMErrSta_enum] -> bus_creator/100
  [VINP_EBMRLampSta_enum] -> bus_creator/101
  [VINP_FrActvDmpDisabSta_flg] -> bus_creator/102
  [VINP_FrEDUDrtSta_flg] -> bus_creator/103
  [VINP_FrEDUOpratingSta_flg] -> bus_creator/104
  [VINP_FrEDURealTMTq_Nm] -> bus_creator/105
  [VINP_FrEDURotateDirction_enum] -> bus_creator/106
  [VINP_FrEDUTqReqFbk_Nm] -> bus_creator/107
  [VINP_FrMCUBAT_V] -> bus_creator/108
  [VINP_FrMCUDCBusCurr_A] -> bus_creator/109
  [VINP_FrMCUDCBusVolt_V] -> bus_creator/110
  [VINP_FrMCUDischrgSta_flg] -> bus_creator/111
  [VINP_FrMCUEnaSta_flg] -> bus_creator/112
  [VINP_FrMCUErr_enum] -> bus_creator/113
  [VINP_FrMCUIGNsta_flg] -> bus_creator/114
  [VINP_FrMCUReady_flg] -> bus_creator/115
  [VINP_FrMCUReady4Pre_flg] -> bus_creator/116
  [VINP_FrMCUSysSta_enum] -> bus_creator/117
  [VINP_FrMCUTemp_C] -> bus_creator/118
  [VINP_FrMotorAvailTq_Nm] -> bus_creator/119
  [VINP_FrRegenAvailTq_Nm] -> bus_creator/120
  [VINP_FrTMSpd_rpm] -> bus_creator/121
  [VINP_FrTMTemp_C] -> bus_creator/122
  [VINP_FrTMid_A] -> bus_creator/123
  [VINP_FrTMiq_A] -> bus_creator/124
  [VINP_MCUWarnF_enum] -> bus_creator/125
  [VINP_MCUBFRealPwrKwSta_kW] -> bus_creator/126
  [VINP_FrCoolanttempReq_C] -> bus_creator/127
  [VINP_FrFailcode1_enum] -> bus_creator/128
  [VINP_FrFailcode2_enum] -> bus_creator/129
  [VINP_FrFailcodehistory1_enum] -> bus_creator/130
  [VINP_FrFailcodehistory2_enum] -> bus_creator/131
  [VINP_FrLLCTemp_C] -> bus_creator/132
  [VINP_FrLLCflowReq_Lpmin] -> bus_creator/133
  [VINP_FrMCUTempWarn_enum] -> bus_creator/134
  [VINP_FrMCUHWVer_enum] -> bus_creator/135
  [VINP_FrMCUSWVer_enum] -> bus_creator/136
  [VINP_FrTMTempWarn_enum] -> bus_creator/137
  [VINP_MCUBFLLCTempWarnSta_enum] -> bus_creator/138
  [VINP_MCUWarnR_enum] -> bus_creator/139
  [VINP_MCUBRRealPwrKwSta_kW] -> bus_creator/140
  [VINP_RrActvDmpDisabSta_flg] -> bus_creator/141
  [VINP_RrEDUDrtSta_flg] -> bus_creator/142
  [VINP_RrEDUOpratingSta_flg] -> bus_creator/143
  [VINP_RrEDURealTMTq_Nm] -> bus_creator/144
  [VINP_RrEDURotateDirction_enum] -> bus_creator/145
  [VINP_RrEDUTqReqFbk_Nm] -> bus_creator/146
  [VINP_RrMCUBAT_V] -> bus_creator/147
  [VINP_RrMCUDCBusCurr_A] -> bus_creator/148
  [VINP_RrMCUDCBusVolt_V] -> bus_creator/149
  [VINP_RrMCUDischrgSta_flg] -> bus_creator/150
  [VINP_RrMCUEnaSta_flg] -> bus_creator/151
  [VINP_RrMCUErr_enum] -> bus_creator/152
  [VINP_RrMCUIGNsta_flg] -> bus_creator/153
  [VINP_RrMCUReady_flg] -> bus_creator/154
  [VINP_RrMCUReady4Pre_flg] -> bus_creator/155
  [VINP_RrMCUSysSta_enum] -> bus_creator/156
  [VINP_RrMCUTemp_C] -> bus_creator/157
  [VINP_RrMotorAvailTq_Nm] -> bus_creator/158
  [VINP_RrRegenAvailTq_Nm] -> bus_creator/159
  [VINP_RrTMSpd_rpm] -> bus_creator/160
  [VINP_RrTMTemp_C] -> bus_creator/161
  [VINP_RrTMid_A] -> bus_creator/162
  [VINP_RrTMiq_A] -> bus_creator/163
  [VINP_MCUBRLLCTempWarnSta_enum] -> bus_creator/164
  [VINP_RrCoolanttempReq_cnt] -> bus_creator/165
  [VINP_RrFailcode1_enum] -> bus_creator/166
  [VINP_RrFailcode2_enum] -> bus_creator/167
  [VINP_RrFailcodehistory1_enum] -> bus_creator/168
  [VINP_RrFailcodehistory2_enum] -> bus_creator/169
  [VINP_RrLLCTemp_C] -> bus_creator/170
  [VINP_RrLLCflowReq_Lpmin] -> bus_creator/171
  [VINP_RrMCU3HWVer_enum] -> bus_creator/172
  [VINP_RrMCU3SWVer_enum] -> bus_creator/173
  [VINP_RrMCUTempWarn_enum] -> bus_creator/174
  [VINP_RrTMTempWarn_enum] -> bus_creator/175
  [VINP_MCUNF1CSErr_flg] -> bus_creator/176
  [VINP_MCUNF1RCErr_flg] -> bus_creator/177
  [VINP_FrActvDmpDisabStaNidec_flg] -> bus_creator/178
  [VINP_FrEDUDrtStaNidec_flg] -> bus_creator/179
  [VINP_FrEDUOpratingStaNidec_flg] -> bus_creator/180
  [VINP_FrEDURealTMTqNidec_Nm] -> bus_creator/181
  [VINP_FrEDURotateDirctionNidec_enum] -> bus_creator/182
  [VINP_FrEDUTqReqFbkNidec_Nm] -> bus_creator/183
  [VINP_FrMCU1ChksumNidec_enum] -> bus_creator/184
  [VINP_FrMCU1RolCntNidec_enum] -> bus_creator/185
  [VINP_FrMCUBATNidec_V] -> bus_creator/186
  [VINP_FrMCUDCBusCurrNidec_A] -> bus_creator/187
  [VINP_FrMCUDCBusVoltNidec_V] -> bus_creator/188
  [VINP_FrMCUDischrgStaNidec_flg] -> bus_creator/189
  [VINP_FrMCUEnaStaNidec_flg] -> bus_creator/190
  [VINP_FrMCUErrNidec_enum] -> bus_creator/191
  [VINP_FrMCUIGNstaNidec_flg] -> bus_creator/192
  [VINP_FrMCUReady4PreNidec_flg] -> bus_creator/193
  [VINP_FrMCUReadyNidec_flg] -> bus_creator/194
  [VINP_FrMCUSysStaNidec_enum] -> bus_creator/195
  [VINP_FrMCUTempNidec_C] -> bus_creator/196
  [VINP_FrMotorAvailTqNidec_Nm] -> bus_creator/197
  [VINP_FrRegenAvailTqNidec_Nm] -> bus_creator/198
  [VINP_FrTMSpdNidec_rpm] -> bus_creator/199
  [VINP_FrTMTempNidec_C] -> bus_creator/200
  [VINP_FrTMidNidec_A] -> bus_creator/201
  [VINP_FrTMiqNidec_A] -> bus_creator/202
  [VINP_MCUWarnFNidec_enum] -> bus_creator/203
  [VINP_FrCoolanttempReqNidec_C] -> bus_creator/204
  [VINP_FrEOPSpdSetNidec_rpm] -> bus_creator/205
  [VINP_FrFailcode1Nidec_enum] -> bus_creator/206
  [VINP_FrFailcode2Nidec_enum] -> bus_creator/207
  [VINP_FrFailcodehistory1Nidec_enum] -> bus_creator/208
  [VINP_FrFailcodehistory2Nidec_enum] -> bus_creator/209
  [VINP_FrLLCTempNidec_C] -> bus_creator/210
  [VINP_FrLLCflowReqNidec_Lpmin] -> bus_creator/211
  [VINP_FrMCUTempWarnNidec_enum] -> bus_creator/212
  [VINP_FrTMTempWarnNidec_enum] -> bus_creator/213
  [VINP_FrMCUHWVerNidec_enum] -> bus_creator/214
  [VINP_FrMCUSWVerNidec_enum] -> bus_creator/215
  [VINP_MCUNR1CSErr_flg] -> bus_creator/216
  [VINP_MCUNR1RCErr_flg] -> bus_creator/217
  [VINP_MCUWarnRNidec_enum] -> bus_creator/218
  [VINP_RrActvDmpDisabStaNidec_flg] -> bus_creator/219
  [VINP_RrEDUDrtStaNidec_flg] -> bus_creator/220
  [VINP_RrEDUOpratingStaNidec_flg] -> bus_creator/221
  [VINP_RrEDURealTMTqNidec_Nm] -> bus_creator/222
  [VINP_RrEDURotateDirctionNidec_enum] -> bus_creator/223
  [VINP_RrEDUTqReqFbkNidec_Nm] -> bus_creator/224
  [VINP_RrMCU1ChksumNidec_enum] -> bus_creator/225
  [VINP_RrMCU1RolCntNidec_enum] -> bus_creator/226
  [VINP_RrMCUBATNidec_V] -> bus_creator/227
  [VINP_RrMCUDCBusCurrNidec_A] -> bus_creator/228
  [VINP_RrMCUDCBusVoltNidec_V] -> bus_creator/229
  [VINP_RrMCUDischrgStaNidec_flg] -> bus_creator/230
  [VINP_RrMCUEnaStaNidec_flg] -> bus_creator/231
  [VINP_RrMCUErrNidec_enum] -> bus_creator/232
  [VINP_RrMCUIGNstaNidec_flg] -> bus_creator/233
  [VINP_RrMCUReady4PreNidec_flg] -> bus_creator/234
  [VINP_RrMCUReadyNidec_flg] -> bus_creator/235
  [VINP_RrMCUSysStaNidec_enum] -> bus_creator/236
  [VINP_RrMCUTempNidec_C] -> bus_creator/237
  [VINP_RrMotorAvailTqNidec_Nm] -> bus_creator/238
  [VINP_RrRegenAvailTqNidec_Nm] -> bus_creator/239
  [VINP_RrTMSpdNidec_rpm] -> bus_creator/240
  [VINP_RrTMTempNidec_C] -> bus_creator/241
  [VINP_RrTMidNidec_A] -> bus_creator/242
  [VINP_RrTMiqNidec_A] -> bus_creator/243
  [VINP_RrCoolanttempReqNidec_cnt] -> bus_creator/244
  [VINP_RrEOPSpdSetNidec_rpm] -> bus_creator/245
  [VINP_RrFailcode1Nidec_enum] -> bus_creator/246
  [VINP_RrFailcode2Nidec_enum] -> bus_creator/247
  [VINP_RrFailcodehistory1Nidec_enum] -> bus_creator/248
  [VINP_RrFailcodehistory2Nidec_enum] -> bus_creator/249
  [VINP_RrLLCTempNidec_C] -> bus_creator/250
  [VINP_RrLLCflowReqNidec_Lpmin] -> bus_creator/251
  [VINP_RrMCUTempWarnNidec_enum] -> bus_creator/252
  [VINP_RrTMTempWarnNidec_enum] -> bus_creator/253
  [VINP_RrMCU3HWVerNidec_enum] -> bus_creator/254
  [VINP_RrMCU3SWVerNidec_enum] -> bus_creator/255
  [VINP_Shifter1CSErr_flg] -> bus_creator/256
  [VINP_Shifter1RCErr_flg] -> bus_creator/257
  [VINP_ShifterCRC8_enum] -> bus_creator/258
  [VINP_ShifterFailsta_enum] -> bus_creator/259
  [VINP_ShifterHandleCmd_enum] -> bus_creator/260
  [VINP_ShifterRC_enum] -> bus_creator/261
  [VINP_Shifter2CSErr_flg] -> bus_creator/262
  [VINP_Shifter2RCErr_flg] -> bus_creator/263
  [VINP_CSW2DimSwSta_flg] -> bus_creator/264
  [VINP_CSW2FWasSwSta_enum] -> bus_creator/265
  [VINP_CSW2FWipSwSta_enum] -> bus_creator/266
  [VINP_CSW2PassSWSta_flg] -> bus_creator/267
  [VINP_CSW2RWipWasSwSta_enum] -> bus_creator/268
  [VINP_CSW2TurnSwSta_enum] -> bus_creator/269

== system inp/INP/CAN4/CommunicationCheck ==
  BHAL_outputs : Inport
  CANMsgInvalidBodyZoneDR1 : FVT_lib/inp/CAN_Msg_Validity_Process_template  SystemSampleTime=-1  VariantActivationTime=update diagram  Latency=0  AutoFrameSizeCalculation=off
      link override ovrdflg: Value=KINP_CANMsgInvalidBodyZoneDR1_flg_ovrdflg
      link override ovrdval: Value=KINP_CANMsgInvalidBodyZoneDR1_flg_ovrdval
  CANMsgInvalidBodyZoneDR2 : FVT_lib/inp/CAN_Msg_Validity_Process_template  SystemSampleTime=-1  VariantActivationTime=update diagram  Latency=0  AutoFrameSizeCalculation=off
      link override ovrdflg: Value=KINP_CANMsgInvalidBodyZoneDR2_flg_ovrdflg
      link override ovrdval: Value=KINP_CANMsgInvalidBodyZoneDR2_flg_ovrdval
  CANMsgInvalidBodyZonePS1 : FVT_lib/inp/CAN_Msg_Validity_Process_template  SystemSampleTime=-1  VariantActivationTime=update diagram  Latency=0  AutoFrameSizeCalculation=off
      link override ovrdflg: Value=KINP_CANMsgInvalidBodyZonePS1_flg_ovrdflg
      link override ovrdval: Value=KINP_CANMsgInvalidBodyZonePS1_flg_ovrdval
  CANMsgInvalidBodyZonePS2 : FVT_lib/inp/CAN_Msg_Validity_Process_template  SystemSampleTime=-1  VariantActivationTime=update diagram  Latency=0  AutoFrameSizeCalculation=off
      link override ovrdflg: Value=KINP_CANMsgInvalidBodyZonePS2_flg_ovrdflg
      link override ovrdval: Value=KINP_CANMsgInvalidBodyZonePS2_flg_ovrdval
  CANMsgInvalidDKC1 : FVT_lib/inp/CAN_Msg_Validity_Process_template  SystemSampleTime=-1  VariantActivationTime=update diagram  Latency=0  AutoFrameSizeCalculation=off
      link override ovrdflg: Value=KINP_CANMsgInvalidDKC1_flg_ovrdflg
      link override ovrdval: Value=KINP_CANMsgInvalidDKC1_flg_ovrdval
  CANMsgInvalidDKC2 : FVT_lib/inp/CAN_Msg_Validity_Process_template  SystemSampleTime=-1  VariantActivationTime=update diagram  Latency=0  AutoFrameSizeCalculation=off
      link override ovrdflg: Value=KINP_CANMsgInvalidDKC2_flg_ovrdflg
      link override ovrdval: Value=KINP_CANMsgInvalidDKC2_flg_ovrdval
  CANMsgInvalidPTG1 : FVT_lib/inp/CAN_Msg_Validity_Process_template  SystemSampleTime=-1  VariantActivationTime=update diagram  Latency=0  AutoFrameSizeCalculation=off
      link override ovrdflg: Value=KINP_CANMsgInvalidPTG1_flg_ovrdflg
      link override ovrdval: Value=KINP_CANMsgInvalidPTG1_flg_ovrdval
  CANMsgInvalidZONEDR1 : FVT_lib/inp/CAN_Msg_Validity_Process_template  SystemSampleTime=-1  VariantActivationTime=update diagram  Latency=0  AutoFrameSizeCalculation=off
      link override ovrdflg: Value=KINP_CANMsgInvalidZONEDR1_flg_ovrdflg
      link override ovrdval: Value=KINP_CANMsgInvalidZONEDR1_flg_ovrdval
  CANMsgInvalidZONEDRVCU : FVT_lib/inp/CAN_Msg_Validity_Process_template  SystemSampleTime=-1  VariantActivationTime=update diagram  Latency=0  AutoFrameSizeCalculation=off
      link override ovrdflg: Value=KINP_CANMsgInvalidZONEDRVCU_flg_ovrdflg
      link override ovrdval: Value=KINP_CANMsgInvalidZONEDRVCU_flg_ovrdval
  CANMsgInvalidZONEFR1 : FVT_lib/inp/CAN_Msg_Validity_Process_template  SystemSampleTime=-1  VariantActivationTime=update diagram  Latency=0  AutoFrameSizeCalculation=off
      link override ovrdflg: Value=KINP_CANMsgInvalidZONEFR1_flg_ovrdflg
      link override ovrdval: Value=KINP_CANMsgInvalidZONEFR1_flg_ovrdval
  CANMsgInvalidZONEFRVCU : FVT_lib/inp/CAN_Msg_Validity_Process_template  SystemSampleTime=-1  VariantActivationTime=update diagram  Latency=0  AutoFrameSizeCalculation=off
      link override ovrdflg: Value=KINP_CANMsgInvalidZONEFRVCU_flg_ovrdflg
      link override ovrdval: Value=KINP_CANMsgInvalidZONEFRVCU_flg_ovrdval
  CANMsgInvalidzGWAPTC1 : FVT_lib/inp/CAN_Msg_Validity_Process_template  SystemSampleTime=-1  VariantActivationTime=update diagram  Latency=0  AutoFrameSizeCalculation=off
      link override ovrdflg: Value=KINP_CANMsgInvalidzGWAPTC1_flg_ovrdflg
      link override ovrdval: Value=KINP_CANMsgInvalidzGWAPTC1_flg_ovrdval
  CANMsgInvalidzGWCANFr1 : FVT_lib/inp/CAN_Msg_Validity_Process_template  SystemSampleTime=-1  VariantActivationTime=update diagram  Latency=0  AutoFrameSizeCalculation=off
      link override ovrdflg: Value=KINP_CANMsgInvalidzGWCANFr1_flg_ovrdflg
      link override ovrdval: Value=KINP_CANMsgInvalidzGWCANFr1_flg_ovrdval
  CANMsgInvalidzGWLINDr1 : FVT_lib/inp/CAN_Msg_Validity_Process_template  SystemSampleTime=-1  VariantActivationTime=update diagram  Latency=0  AutoFrameSizeCalculation=off
      link override ovrdflg: Value=KINP_CANMsgInvalidzGWLINDr1_flg_ovrdflg
      link override ovrdval: Value=KINP_CANMsgInvalidzGWLINDr1_flg_ovrdval
  CANMsgInvalidzGWLINDr2 : FVT_lib/inp/CAN_Msg_Validity_Process_template  SystemSampleTime=-1  VariantActivationTime=update diagram  Latency=0  AutoFrameSizeCalculation=off
      link override ovrdflg: Value=KINP_CANMsgInvalidzGWLINDr2_flg_ovrdflg
      link override ovrdval: Value=KINP_CANMsgInvalidzGWLINDr2_flg_ovrdval
  CANMsgInvalidzGWLINFr1 : FVT_lib/inp/CAN_Msg_Validity_Process_template  SystemSampleTime=-1  VariantActivationTime=update diagram  Latency=0  AutoFrameSizeCalculation=off
      link override ovrdflg: Value=KINP_CANMsgInvalidzGWLINFr1_flg_ovrdflg
      link override ovrdval: Value=KINP_CANMsgInvalidzGWLINFr1_flg_ovrdval
  CANMsgInvalidzGWLINFr2 : FVT_lib/inp/CAN_Msg_Validity_Process_template  SystemSampleTime=-1  VariantActivationTime=update diagram  Latency=0  AutoFrameSizeCalculation=off
      link override ovrdflg: Value=KINP_CANMsgInvalidzGWLINFr2_flg_ovrdflg
      link override ovrdval: Value=KINP_CANMsgInvalidzGWLINFr2_flg_ovrdval
  CANMsgInvalidzGWSEAT1 : FVT_lib/inp/CAN_Msg_Validity_Process_template  SystemSampleTime=-1  VariantActivationTime=update diagram  Latency=0  AutoFrameSizeCalculation=off
      link override ovrdflg: Value=KINP_CANMsgInvalidzGWSEAT1_flg_ovrdflg
      link override ovrdval: Value=KINP_CANMsgInvalidzGWSEAT1_flg_ovrdval
  bus_creator : BusCreator  Inputs=18
  bus_selector : BusSelector  OutputSignals=VHAL_CANMsgInvalidBodyZoneDR1_flg,VHAL_CANMsgInvalidBodyZoneDR2_flg,VHAL_CANMsgInvalidBodyZonePS1_flg,VHAL_CANMsgInvalidBodyZonePS2_flg,VHAL_CANMsgInvalidDKC1_flg,VHAL_CANMsgInvalidDKC2_flg,VHAL_CANMsgInvalidPTG1_flg,VHAL_CANMsgInvalidZONEDR1_flg,VHAL_CANMsgInvalidZONEDRVCU_flg,VHAL_CANMsgInvalidZONEFR1_flg,VHAL_CANMsgInvalidZONEFRVCU_flg,VHAL_CANMsgInvalidzGWAPTC1_flg,VHAL_CANMsgInvalidzGWCANFr1_flg,VHAL_CANMsgInvalidzGWLINDr1_flg,VHAL_CANMsgInvalidzGWLINDr2_flg,VHAL_CANMsgInvalidzGWLINFr1_flg,VHAL_CANMsgInvalidzGWLINFr2_flg,VHAL_CANMsgInvalidzGWSEAT1_flg
  not{1..18} (18 alike) : Logic  Operator=NOT  AllPortsSameDT=off  OutDataTypeStr=boolean
  inp_CanValid_bus : Outport
  wires:
  BHAL_outputs/1 -> [BHAL_outputs]
  bus_selector/1 -> CANMsgInvalidBodyZoneDR1/1  "<VHAL_CANMsgInvalidBodyZoneDR1_flg>"
  CANMsgInvalidBodyZoneDR1/1 -> not1/1
  not1/1 -> bus_creator/1  "VINP_CANMsgValidBodyZoneDR1_flg"
  bus_selector/2 -> CANMsgInvalidBodyZoneDR2/1  "<VHAL_CANMsgInvalidBodyZoneDR2_flg>"
  CANMsgInvalidBodyZoneDR2/1 -> not2/1
  not2/1 -> bus_creator/2  "VINP_CANMsgValidBodyZoneDR2_flg"
  bus_selector/3 -> CANMsgInvalidBodyZonePS1/1  "<VHAL_CANMsgInvalidBodyZonePS1_flg>"
  CANMsgInvalidBodyZonePS1/1 -> not3/1
  not3/1 -> bus_creator/3  "VINP_CANMsgValidBodyZonePS1_flg"
  bus_selector/4 -> CANMsgInvalidBodyZonePS2/1  "<VHAL_CANMsgInvalidBodyZonePS2_flg>"
  CANMsgInvalidBodyZonePS2/1 -> not4/1
  not4/1 -> bus_creator/4  "VINP_CANMsgValidBodyZonePS2_flg"
  bus_selector/5 -> CANMsgInvalidDKC1/1  "<VHAL_CANMsgInvalidDKC1_flg>"
  CANMsgInvalidDKC1/1 -> not5/1
  not5/1 -> bus_creator/5  "VINP_CANMsgValidDKC1_flg"
  bus_selector/6 -> CANMsgInvalidDKC2/1  "<VHAL_CANMsgInvalidDKC2_flg>"
  CANMsgInvalidDKC2/1 -> not6/1
  not6/1 -> bus_creator/6  "VINP_CANMsgValidDKC2_flg"
  bus_selector/7 -> CANMsgInvalidPTG1/1  "<VHAL_CANMsgInvalidPTG1_flg>"
  CANMsgInvalidPTG1/1 -> not7/1
  not7/1 -> bus_creator/7  "VINP_CANMsgValidPTG1_flg"
  bus_selector/8 -> CANMsgInvalidZONEDR1/1  "<VHAL_CANMsgInvalidZONEDR1_flg>"
  CANMsgInvalidZONEDR1/1 -> not8/1
  not8/1 -> bus_creator/8  "VINP_CANMsgValidZONEDR1_flg"
  bus_selector/9 -> CANMsgInvalidZONEDRVCU/1  "<VHAL_CANMsgInvalidZONEDRVCU_flg>"
  CANMsgInvalidZONEDRVCU/1 -> not9/1
  not9/1 -> bus_creator/9  "VINP_CANMsgValidZONEDRVCU_flg"
  bus_selector/10 -> CANMsgInvalidZONEFR1/1  "<VHAL_CANMsgInvalidZONEFR1_flg>"
  CANMsgInvalidZONEFR1/1 -> not10/1
  not10/1 -> bus_creator/10  "VINP_CANMsgValidZONEFR1_flg"
  bus_selector/11 -> CANMsgInvalidZONEFRVCU/1  "<VHAL_CANMsgInvalidZONEFRVCU_flg>"
  CANMsgInvalidZONEFRVCU/1 -> not11/1
  not11/1 -> bus_creator/11  "VINP_CANMsgValidZONEFRVCU_flg"
  bus_selector/12 -> CANMsgInvalidzGWAPTC1/1  "<VHAL_CANMsgInvalidzGWAPTC1_flg>"
  CANMsgInvalidzGWAPTC1/1 -> not12/1
  not12/1 -> bus_creator/12  "VINP_CANMsgValidzGWAPTC1_flg"
  bus_selector/13 -> CANMsgInvalidzGWCANFr1/1  "<VHAL_CANMsgInvalidzGWCANFr1_flg>"
  CANMsgInvalidzGWCANFr1/1 -> not13/1
  not13/1 -> bus_creator/13  "VINP_CANMsgValidzGWCANFr1_flg"
  bus_selector/14 -> CANMsgInvalidzGWLINDr1/1  "<VHAL_CANMsgInvalidzGWLINDr1_flg>"
  CANMsgInvalidzGWLINDr1/1 -> not14/1
  not14/1 -> bus_creator/14  "VINP_CANMsgValidzGWLINDr1_flg"
  bus_selector/15 -> CANMsgInvalidzGWLINDr2/1  "<VHAL_CANMsgInvalidzGWLINDr2_flg>"
  CANMsgInvalidzGWLINDr2/1 -> not15/1
  not15/1 -> bus_creator/15  "VINP_CANMsgValidzGWLINDr2_flg"
  bus_selector/16 -> CANMsgInvalidzGWLINFr1/1  "<VHAL_CANMsgInvalidzGWLINFr1_flg>"
  CANMsgInvalidzGWLINFr1/1 -> not16/1
  not16/1 -> bus_creator/16  "VINP_CANMsgValidzGWLINFr1_flg"
  bus_selector/17 -> CANMsgInvalidzGWLINFr2/1  "<VHAL_CANMsgInvalidzGWLINFr2_flg>"
  CANMsgInvalidzGWLINFr2/1 -> not17/1
  not17/1 -> bus_creator/17  "VINP_CANMsgValidzGWLINFr2_flg"
  bus_selector/18 -> CANMsgInvalidzGWSEAT1/1  "<VHAL_CANMsgInvalidzGWSEAT1_flg>"
  CANMsgInvalidzGWSEAT1/1 -> not18/1
  not18/1 -> bus_creator/18  "VINP_CANMsgValidzGWSEAT1_flg"
  [BHAL_outputs] -> bus_selector/1
  bus_creator/1 -> inp_CanValid_bus/1
